simulink model "filter_1_10_2"  (Simulink 7.8)
settings: Solver=ode45  StartTime=0.0  StopTime=10  RelTol=1e-3
libraries: dsparch4 x8, dspsigops x6
settings Model: Creator=svenhoffmann  LastModifiedBy=josef  ExtModeAutoUpdateStatusClock=off
settings DataIOCC: SignalLoggingName=sigsOut
settings OptimizationCC: InitFltsAndDblsToZero=on
settings DebuggingCC: SaveWithParameterizedLinksMsg=none  SignalResolutionControl=TryResolveAllWithWarning  SolverPrmCheckMsg=none  MultiTaskDSMMsg=warning  MultiTaskCondExecSysMsg=none  FcnCallInpInsideContextMsg=Use local settings  StrictBusMsg=None
settings HardwareCC: TargetUnknown=on
settings RTWCC: IncludeERTFirstTime=on
settings GRTTargetCC: TargetFcnLib=ansi_tfl_tmw.mat

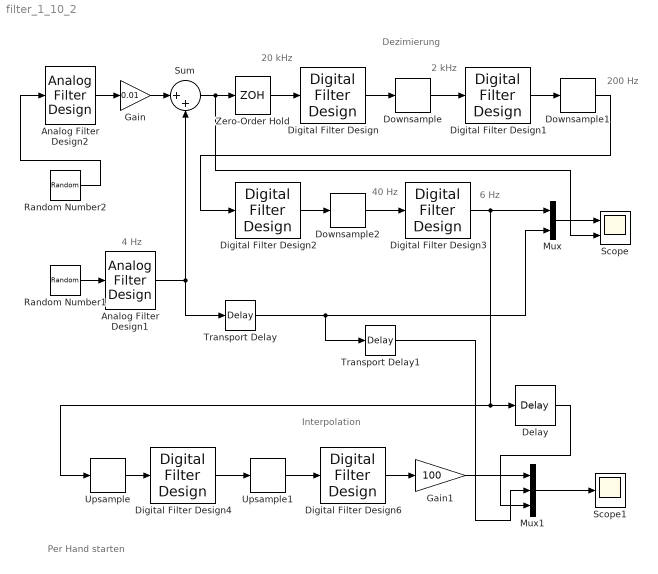
== system filter_1_10_2 ==
  note: 20 kHz
  note: 2 kHz
  note: 200 Hz
  note: 40 Hz
  note: 6 Hz
  note: 4 Hz
  note: Interpolation
  note: Dezimierung
  note: Per Hand starten
  Analog Filter Design1 : dsparch4/Analog Filter Design  method=Chebyshev I  filttype=Lowpass  N=8  Wlo=2*pi*4  Whi=2*pi*4000  Rp=2  Rs=40
  Analog Filter Design2 : dsparch4/Analog Filter Design  method=Chebyshev I  filttype=Bandpass  N=8  Wlo=2*pi*100  Whi=2*pi*4000  Rp=2  Rs=40
  Delay : dspsigops/Delay  InputProcessing=Inherited (this choice will be removed - see release notes)  dly_unit=Samples  delay=10  ic_detail=off  dif_ic_for_ch=off  dif_ic_for_dly=off  ic=0  reset_popup=None
  Digital Filter Design{,1..4,6} (6 alike) : dsparch4/Digital Filter Design  mwdsp_browser_bugfix_var=off
  Downsample : dspsigops/Downsample  N=10  phase=0  InputProcessing=Inherited (this choice will be removed - see release notes)  RateOptions=Enforce single-rate processing  smode=Allow multirate  fmode=Maintain input frame size  ic=0
  Downsample1 : dspsigops/Downsample  N=10  phase=0  InputProcessing=Inherited (this choice will be removed - see release notes)  RateOptions=Enforce single-rate processing  smode=Allow multirate  fmode=Maintain input frame size  ic=0
  Downsample2 : dspsigops/Downsample  N=5  phase=0  InputProcessing=Inherited (this choice will be removed - see release notes)  RateOptions=Enforce single-rate processing  smode=Allow multirate  fmode=Maintain input frame size  ic=0
  Gain : Gain  Gain=0.01  SaturateOnIntegerOverflow=on  OutDataTypeStr=Inherit: Same as input  ParamDataTypeStr=Inherit: Same as input
  Gain1 : Gain  Gain=100  SaturateOnIntegerOverflow=on  OutDataTypeStr=Inherit: Same as input  ParamDataTypeStr=Inherit: Same as input
  Mux : Mux  Inputs=2
  Mux1 : Mux  Inputs=3
  Random Number1 : RandomNumber  Seed=1375  SampleTime=0
  Random Number2 : RandomNumber  SampleTime=0
  Scope : Scope  NumInputPorts=2
      settings: TimeRange=2  YMin=-0.05~-0.15  YMax=0.055~0.15  MaxDataPoints=20000
  Scope1 : Scope
      settings: TimeRange=2  YMin=-0.055  YMax=0.05  MaxDataPoints=20000
  Sum : Sum  Inputs=|++  SaturateOnIntegerOverflow=on
  Transport Delay : TransportDelay  DelayTime=0.17  BufferSize=2048
  Transport Delay1 : TransportDelay  DelayTime=0.245  BufferSize=2048
  Upsample : dspsigops/Upsample  N=10  phase=0  InputProcessing=Inherited (this choice will be removed - see release notes)  RateOptions=Allow multirate processing  ic=0  mode=Unused parameter value
  Upsample1 : dspsigops/Upsample  N=10  phase=0  InputProcessing=Inherited (this choice will be removed - see release notes)  RateOptions=Allow multirate processing  ic=0  mode=Unused parameter value
  Zero-Order Hold : ZeroOrderHold  SampleTime=1/20000
  wires:
  Analog Filter Design1/1 -> Sum/2, Transport Delay/1
  Random Number2/1 -> Analog Filter Design2/1
  Analog Filter Design2/1 -> Gain/1
  Gain/1 -> Sum/1
  Sum/1 -> Zero-Order Hold/1, Scope/2
  Digital Filter Design/1 -> Downsample/1
  Downsample/1 -> Digital Filter Design1/1
  Digital Filter Design1/1 -> Downsample1/1
  Digital Filter Design2/1 -> Downsample2/1
  Downsample1/1 -> Digital Filter Design2/1
  Zero-Order Hold/1 -> Digital Filter Design/1
  Downsample2/1 -> Digital Filter Design3/1
  Digital Filter Design3/1 -> Mux/1, Delay/1, Upsample/1
  Mux/1 -> Scope/1
  Transport Delay/1 -> Mux/2, Transport Delay1/1
  Random Number1/1 -> Analog Filter Design1/1
  Upsample/1 -> Digital Filter Design4/1
  Upsample1/1 -> Digital Filter Design6/1
  Digital Filter Design4/1 -> Upsample1/1
  Gain1/1 -> Mux1/1
  Transport Delay1/1 -> Mux1/2
  Delay/1 -> Mux1/3
  Mux1/1 -> Scope1/1
  Digital Filter Design6/1 -> Gain1/1
